simulink model "lr6"  (R2024a)
settings: Solver=VariableStepAuto  StartTime=0.0  StopTime=0.2  MaxStep=1e-4  RelTol=1e-5
undefined symbols (not defined in the file): DC_voltage, freq_mod, koef_mod, Kratnost_NesMod, Nagr, U_f, U_fd
libraries: spsFourierLib x4, spsCurrentMeasurementLib x2, spsVoltageMeasurementLib x2, spsDCVoltageSourceLib x1, spsMultimeterLib x1, spsPWMGenerator2LevelLib x1, spsRMSLib x1, spsThreePhaseSeriesRLCBranchLib x1, spsUniversalBridgeLib x1, sps_lib x1
settings Model: Creator=Руслан  LastModifiedBy=79532
settings DataIOCC: SaveFormat=StructureWithTime  ReturnWorkspaceOutputs=off

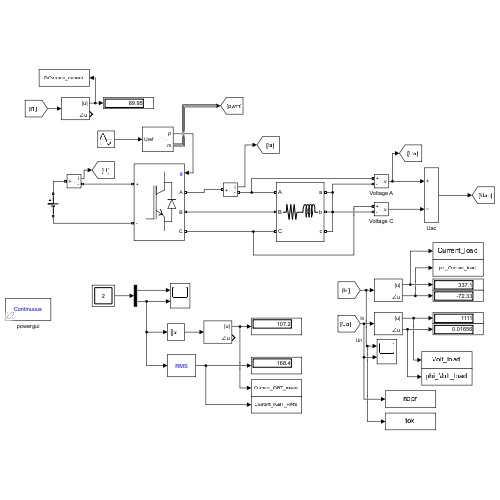
[thumbnail: Simulink's stored preview of the top-level diagram]
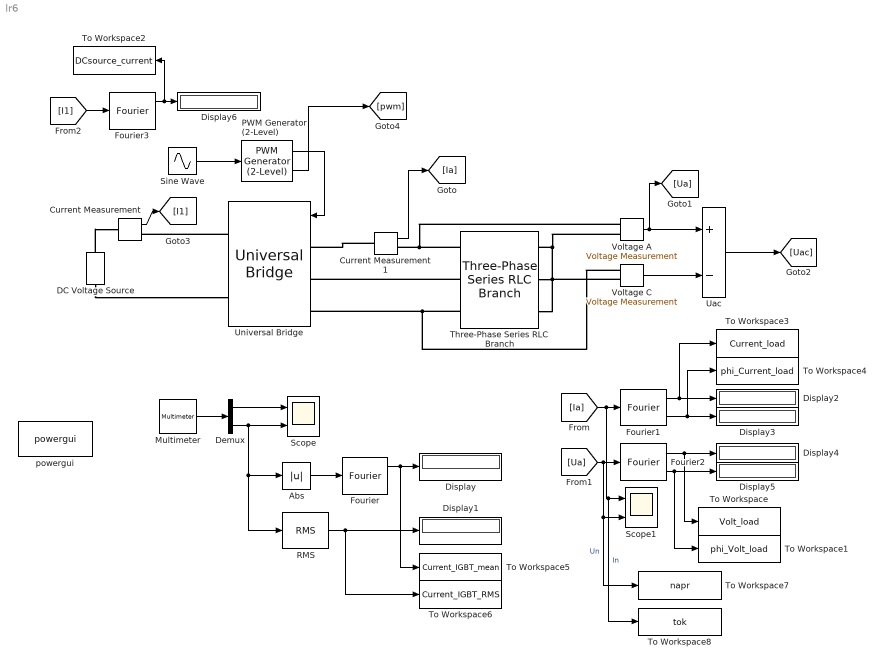
== system lr6 ==
  Abs : Abs  SaturateOnIntegerOverflow=off
  Current Measurement : spsCurrentMeasurementLib/Current Measurement  PhasorSimulation=off  OutputType=Complex  PSBequivalent=0
  Current Measurement1 : spsCurrentMeasurementLib/Current Measurement  PhasorSimulation=off  OutputType=Complex  PSBequivalent=0
  DC Voltage Source : spsDCVoltageSourceLib/DC Voltage Source  Amplitude=DC_voltage  Measurements=None
  Demux : Demux  Outputs=2
  Display{,1..6} (7 alike) : Display
  Fourier : spsFourierLib/Fourier  Freq=freq_mod  n=0  InInit=[0, 0]  Ts=0
  Fourier1 : spsFourierLib/Fourier  Freq=freq_mod  n=1  InInit=[0, 0]  Ts=0
  Fourier2 : spsFourierLib/Fourier  Freq=freq_mod  n=1  InInit=[0, 0]  Ts=0
  Fourier3 : spsFourierLib/Fourier  Freq=freq_mod  n=0  InInit=[0, 0]  Ts=0
  Multimeter : spsMultimeterLib/Multimeter  L=16  sel=[1 11]  yselected={}  Gain=[1 1]  OutputType=Complex  PlotAtSimulationStop=off  PhasorSimulation=off
  PWM Generator (2-Level) : spsPWMGenerator2LevelLib/PWM Generator (2-Level)  ModulatorType=Three-phase bridge (6 pulses)  ModulatorMode=Unsynchronized  Fc=freq_mod*Kratnost_NesMod  Pc=90  nF=27  MinMax="[ -1  1 ]"  SamplingTechnique=Natural  ModulatingSignals=off  m=0.8  Freq=60  Phase=0  Ts=0  ShowCarrierOutport=on
  RMS : spsRMSLib/RMS  TrueRMS=on  Freq=freq_mod  RMSInit=0  Ts=0
  Scope : Scope  NumInputPorts=2
  Scope1 : Scope  NumInputPorts=2
  Sine Wave : Sin  Amplitude=koef_mod  Frequency=2*pi*freq_mod  Phase=[0 -2*pi/3 2*pi/3]  SampleTime=0
  Three-Phase Series RLC Branch : spsThreePhaseSeriesRLCBranchLib/Three-Phase Series RLC Branch  LConnTagsString=A|B|C  RConnTagsString=A|B|C  BranchType=RL  Resistance=Nagr.Res  Inductance=Nagr.Ind  Capacitance=1e-6  Measurements=None
  To Workspace : ToWorkspace  VariableName=Volt_load  SampleTime=-1
  To Workspace1 : ToWorkspace  VariableName=phi_Volt_load  SampleTime=-1
  To Workspace2 : ToWorkspace  VariableName=DCsource_current  SampleTime=-1
  To Workspace3 : ToWorkspace  VariableName=Current_load  SampleTime=-1
  To Workspace4 : ToWorkspace  VariableName=phi_Current_load  SampleTime=-1
  To Workspace5 : ToWorkspace  VariableName=Current_IGBT_mean  SampleTime=-1
  To Workspace6 : ToWorkspace  VariableName=Current_IGBT_RMS  SampleTime=-1
  To Workspace7 : ToWorkspace  VariableName=napr  SaveFormat=Timeseries  SampleTime=0.00001
      settings: MaxDataPoints=10000
  To Workspace8 : ToWorkspace  VariableName=tok  SaveFormat=Timeseries  SampleTime=0.00001
      settings: MaxDataPoints=10000
  Uac : Sum  Inputs=+-
  Universal Bridge : spsUniversalBridgeLib/Universal Bridge  Arms=3  SnubberResistance=1e5  SnubberCapacitance=inf  Device=IGBT / Diodes  Ron=R_on  Lon=0  ForwardVoltages="[  U_f  U_fd  ]"  ForwardVoltage=0  GTOparameters=[ 10e-6 , 20e-6 ]  IGBTparameters=[ 1e-6 , 2e-6 ]  Measurements=All voltages and currents  Measurements_2=None  converterType=Rectifier
  Voltage A : spsVoltageMeasurementLib/Voltage Measurement  PhasorSimulation=off  OutputType=Complex  PSBequivalent=0
  Voltage C : spsVoltageMeasurementLib/Voltage Measurement  PhasorSimulation=off  OutputType=Complex  PSBequivalent=0
  powergui : sps_lib/powergui  Priority=1  SimulationMode=Continuous  SampleTime=50e-6  frequency=60  Iterations=50  frequencyindice=0  Pbase=100e6  ErrMax=1e-4  UnitsV=kV  UnitsW=MW  buscounter=0  FunctionMessages=off  echomessages=off  EnableUseOfTLC=off  CurrentSourceSwitches=off  DisableSnubberDevices=off  DisableRonSwitches=off  DisableVfSwitches=off  DisplayEquations=off  AutomaticDiscreteSolvers=off  SolverType=Tustin/Backward Euler (TBE)  Interpol=off  ExternalGateDelay=off  methode=off  Ts=100  x0status=blocks  SPID=on  SwTol=0  HookPort=off  NonlinearTolerance=1e-4  nMaxIteration=100  ContinueOnMaxIteration=off  RestoreLinks=warning  ResistiveCurrentMeasurement=off  Frange=[0:2:500]  Ylog=off  Xlog=on  ShowGrid=off  save=off  variable=ZData  structure=0  ZoomFFT=off  StartTime=0.0  cycles=1  DisplayStyle=1  fundamental=60  FreqAxis=off  MaxFrequency=1000  frequencyindicesteady=1  RmsSteady=1  display=off
  wires:
  Voltage A/1 -> [Ua], Uac/1
  Voltage C/1 -> Uac/2
  Sine Wave/1 -> PWM Generator (2-Level)/1
  PWM Generator (2-Level)/1 -> Universal Bridge/1
  Multimeter/1 -> Demux/1
  Demux/1 -> Scope/1
  Demux/2 -> Abs/1, RMS/1, Scope/2
  Abs/1 -> Fourier/1
  Fourier/1 -> To Workspace5/1, Display/1
  RMS/1 -> To Workspace6/1, Display1/1
  Current Measurement1/1 -> [Ia]
  [Ia] -> To Workspace8/1, Scope1/1, Fourier1/1  "In"
  Fourier1/1 -> To Workspace3/1, Display2/1
  Fourier1/2 -> To Workspace4/1, Display3/1
  Fourier2/2 -> To Workspace1/1, Display5/1
  Fourier2/1 -> To Workspace/1, Display4/1
  [Ua] -> To Workspace7/1, Scope1/2, Fourier2/1  "Un"
  Uac/1 -> [Uac]
  Current Measurement/1 -> [I1]
  PWM Generator (2-Level)/2 -> [pwm]
  Fourier3/1 -> To Workspace2/1, Display6/1
  [I1] -> Fourier3/1
  connections:
  Universal Bridge/RConn1 -- Current Measurement/RConn1
  DC Voltage Source/RConn1 -- Current Measurement/LConn1
  DC Voltage Source/LConn1 -- Universal Bridge/RConn2
  Current Measurement1/LConn1 -- Universal Bridge/LConn1
  Three-Phase Series RLC Branch/LConn2 -- Universal Bridge/LConn2
  Three-Phase Series RLC Branch/LConn3 -- Voltage C/LConn1 -- Universal Bridge/LConn3
  Three-Phase Series RLC Branch/RConn3 -- Voltage C/LConn2 -- Three-Phase Series RLC Branch/RConn2 -- Voltage A/LConn2 -- Three-Phase Series RLC Branch/RConn1
  Three-Phase Series RLC Branch/LConn1 -- Voltage A/LConn1 -- Current Measurement1/RConn1
